simulink model "control"  (R2024a)
settings: Solver=VariableStepAuto  StartTime=0.0  StopTime=4.5  RelTol=1e-3
values from neighbouring files (symbols this model uses):
  params = [m1; m2; a1; a2; kj1; kj2; lbz-rj1; ac1; ac2]    [init_mpc.m]    (also in init_mpc_EKF.m; init_mpc_constraint.m; stateFcnRoboticArmEKF.m = uk(3:11))
libraries: mpclib x1, SignalEditorBlockLib x1
settings Model: Creator=berto  LastModifiedBy=berto

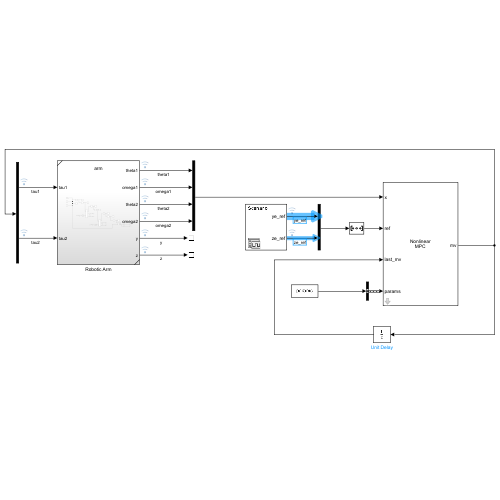
[thumbnail: Simulink's stored preview of the top-level diagram]
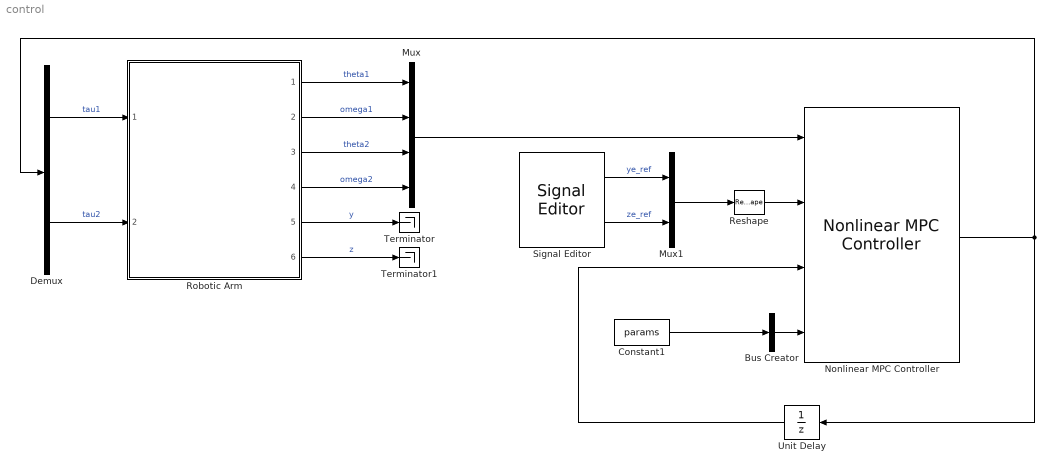
== system control ==
  Bus Creator : BusCreator  Inputs=1  OutDataTypeStr=Bus: paramsBusObject  NonVirtualBus=on
      settings: InheritFromInputs=off
  Constant1 : Constant  Value=params
  Demux : Demux  Outputs=2
  Mux : Mux
  Mux1 : Mux  Inputs=2
  Nonlinear MPC Controller : mpclib/Nonlinear MPC Controller  nlmpcobj=nlobj  UseObjectTs=on  UseMEX=off  md_enabled=off  mvtarget_enabled=off  param_enabled=on  cost_enabled=off  mvseq_enabled=off  stateseq_enabled=off  ovseq_enabled=off  slack_enabled=off  status_enabled=off  ov_min=off  ov_max=off  mv_min=off  mv_max=off  mvrate_min=off  mvrate_max=off  state_min=off  state_max=off  ov_weight=off  mv_weight=off  mvrate_weight=off  ecr_weight=off  nlp_initialize=off
  Reshape : Reshape  OutputDimensionality=Row vector (2-D)
  Robotic Arm : Subsystem  ReferencedSubsystem=arm
  Signal Editor : SignalEditorBlockLib/Signal Editor  FileName=ref.mat  ActiveScenario=Scenario  ActiveSignal=ye_ref  IsBus=off  OutputBusObjectStr=Bus: BusObject  SampleTime=0  Interpolate=off  ZeroCross=off  OutputAfterFinalValue=Setting to zero  Unit=inherit  PreserveSignalName=on  ApplySigPropsToAllScenarios=on  ApplySigPropsToAllSignals=off
  Terminator : Terminator
  Terminator1 : Terminator
  Unit Delay : UnitDelay  SampleTime=-1  HasFrameUpgradeWarning=on
  wires:
  Robotic Arm/1 -> Mux/1  "theta1"
  Robotic Arm/3 -> Mux/3  "theta2"
  Robotic Arm/2 -> Mux/2  "omega1"
  Robotic Arm/4 -> Mux/4  "omega2"
  Mux/1 -> Nonlinear MPC Controller/1
  Nonlinear MPC Controller/1 -> Unit Delay/1, Demux/1
  Unit Delay/1 -> Nonlinear MPC Controller/3
  Demux/1 -> Robotic Arm/1  "tau1"
  Demux/2 -> Robotic Arm/2  "tau2"
  Constant1/1 -> Bus Creator/1
  Bus Creator/1 -> Nonlinear MPC Controller/4
  Reshape/1 -> Nonlinear MPC Controller/2
  Robotic Arm/5 -> Terminator/1  "y"
  Robotic Arm/6 -> Terminator1/1  "z"
  Signal Editor/1 -> Mux1/1  "ye_ref"
  Signal Editor/2 -> Mux1/2  "ze_ref"
  Mux1/1 -> Reshape/1
